simulink model "RCAMSimulation"  (R2020b)
settings: Solver=VariableStepAuto  StartTime=0.0  StopTime=TF  RelTol=1e-3
values from neighbouring files (symbols this model uses):
  u1max = 25*pi/180    (= 0.436332312999)    [InitializeConstants.m]
  u1min = -25*pi/180    (= -0.436332312999)    [InitializeConstants.m]
  u2max = 10*pi/180    (= 0.174532925199)    [InitializeConstants.m]
  u2min = -25*pi/180    (= -0.436332312999)    [InitializeConstants.m]
  u3max = 30*pi/180    (= 0.523598775598)    [InitializeConstants.m]
  u3min = -30*pi/180    (= -0.523598775598)    [InitializeConstants.m]
  u4max = 10*pi/180    (= 0.174532925199)    [InitializeConstants.m]
  u4min = 0.5*pi/180    (= 0.00872664625997)    [InitializeConstants.m]
  u5max = 10*pi/180    (= 0.174532925199)    [InitializeConstants.m]
  u5min = 0.5*pi/180    (= 0.00872664625997)    [InitializeConstants.m]
  x0 = [85 ... (first row only)    [InitializeConstants.m]
undefined symbols (not defined in the file or in its folder): Earth, RCAM_model, WGS84
libraries: aerolibutil x2, aerolibtransform2 x1, aerolibfltsims x1, vrlib x1
settings Model: Creator=admin  LastModifiedBy=Markus

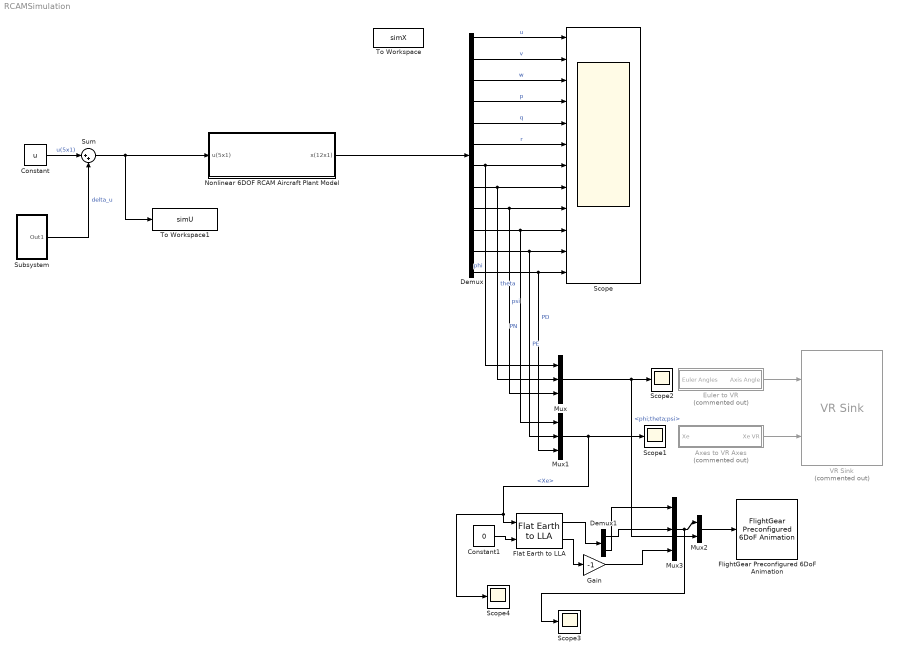
== system RCAMSimulation ==
  Axes to VR Axes : Subsystem  Commented=on
  Constant : Constant  Value=u
  Constant1 : Constant  Value=0
  Demux : Demux  Outputs=12
  Demux1 : Demux  Outputs=2
  Euler to VR : Subsystem  Commented=on
  Flat Earth to LLA : aerolibtransform2/Flat Earth to LLA  units=Metric (MKS)  ptype=Earth (WGS84)  F=1/298.257223563  R=6378137  refPosPort=off  LL0=[0 10]  psi=0
  FlightGear Preconfigured 6DoF Animation : aerolibfltsims/FlightGear Preconfigured 6DoF Animation  xFlightGearVersion=v2019.1  DestinationIpAddress=127.0.0.1  DestinationPort=5502  SampleTime=1/30  packetVersion=24
  Gain : Gain  Gain=-1
  Mux : Mux  Inputs=3
  Mux1 : Mux  Inputs=3
  Mux2 : Mux  Inputs=2
  Mux3 : Mux  Inputs=3
  Nonlinear 6DOF RCAM Aircraft Plant Model : Subsystem
  Scope : Scope  NumInputPorts=12
  Scope{1..4} (4 alike) : Scope
  Subsystem : Subsystem
  Sum : Sum  Inputs=|++
  To Workspace : ToWorkspace  VariableName=simX  SaveFormat=Timeseries  SampleTime=-1
  To Workspace1 : ToWorkspace  VariableName=simU  SaveFormat=Timeseries  SampleTime=-1
  VR Sink : vrlib/VR Sink  Commented=on  InstantiateOnLoad=on  SampleTime=0.1  ViewEnable=on  RemoteChange=off  RemoteView=off  FieldsWritten=HL20.rotation.4.1.1.double#HL20.translation.3.1.1.double  WorldFileName=aeroblk_HL20.wrl  WorldDescription=aeroblk_HL20  AutoView=on  VideoDimensions=[]  AllowVariableSize=off
  wires:
  Nonlinear 6DOF RCAM Aircraft Plant Model/1(x(12x1)) -> Demux/1
  Constant/1 -> Sum/1  "u(5x1)"
  Subsystem/1(Out1) -> Sum/2  "delta_u"
  Sum/1 -> To Workspace1/1, Nonlinear 6DOF RCAM Aircraft Plant Model/1(u(5x1))
  Demux/1 -> Scope/1  "u"
  Demux/2 -> Scope/2  "v"
  Demux/3 -> Scope/3  "w"
  Demux/4 -> Scope/4  "p"
  Demux/5 -> Scope/5  "q"
  Demux/6 -> Scope/6  "r"
  Demux/7 -> Mux/1, Scope/7  "phi"
  Demux/8 -> Mux/2, Scope/8  "theta"
  Demux/9 -> Mux/3, Scope/9  "psi"
  Demux/10 -> Mux1/1, Scope/10  "PN"
  Demux/11 -> Mux1/2, Scope/11  "PE"
  Demux/12 -> Mux1/3, Scope/12  "PD"
  Euler to VR/1(Axis Angle) -> VR Sink/1
  Mux1/1 -> Scope4/1, Flat Earth to LLA/1, Scope1/1  "<Xe>"
  Axes to VR Axes/1(Xe VR) -> VR Sink/2
  Mux/1 -> Mux2/2, Scope2/1  "<phi;theta;psi>"
  Constant1/1 -> Flat Earth to LLA/2
  Mux2/1 -> FlightGear Preconfigured 6DoF Animation/1
  Flat Earth to LLA/1 -> Demux1/1
  Mux3/1 -> Scope3/1, Mux2/1
  Demux1/1 -> Mux3/2
  Flat Earth to LLA/2 -> Gain/1
  Demux1/2 -> Mux3/1
  Gain/1 -> Mux3/3

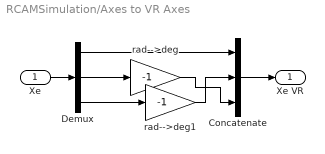
== system RCAMSimulation/Axes to VR Axes ==
  Xe : Inport
  Concatenate : Concatenate  NumInputs=3
  Demux : Demux  Outputs=3
      settings: DisplayOption=none
  rad-->deg : Gain  Gain=-1  SaturateOnIntegerOverflow=on  OutDataTypeStr=Inherit: Same as input  ParamDataTypeStr=Inherit: Same as input
  rad-->deg1 : Gain  Gain=-1  SaturateOnIntegerOverflow=on  OutDataTypeStr=Inherit: Same as input  ParamDataTypeStr=Inherit: Same as input
  Xe VR : Outport  VectorParamsAs1DForOutWhenUnconnected=off
  wires:
  Xe/1 -> Demux/1
  Demux/1 -> Concatenate/1
  Demux/2 -> rad-->deg/1
  Demux/3 -> rad-->deg1/1
  Concatenate/1 -> Xe VR/1
  rad-->deg1/1 -> Concatenate/2
  rad-->deg/1 -> Concatenate/3

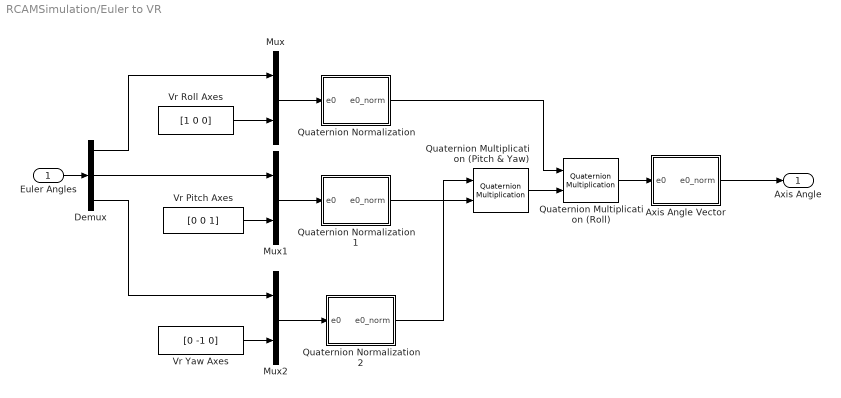
== system RCAMSimulation/Euler to VR ==
  Euler Angles : Inport
  Axis Angle Vector : Subsystem
  Demux : Demux  Outputs=3
      settings: DisplayOption=none
  Mux : Mux  Inputs=2
  Mux1 : Mux  Inputs=2
  Mux2 : Mux  Inputs=2
  Quaternion Multiplication (Pitch & Yaw) : aerolibutil/Quaternion Multiplication
  Quaternion Multiplication (Roll) : aerolibutil/Quaternion Multiplication
  Quaternion Normalization : Subsystem
  Quaternion Normalization1 : Subsystem
  Quaternion Normalization2 : Subsystem
  Vr Pitch Axes : Constant  Value=[0 0 1]
  Vr Roll Axes : Constant  Value=[1 0 0]
  Vr Yaw Axes : Constant  Value=[0 -1 0]
  Axis Angle : Outport  VectorParamsAs1DForOutWhenUnconnected=off
  wires:
  Quaternion Multiplication (Roll)/1 -> Axis Angle Vector/1(e0)
  Quaternion Multiplication (Pitch & Yaw)/1 -> Quaternion Multiplication (Roll)/2
  Axis Angle Vector/1(e0_norm) -> Axis Angle/1
  Quaternion Normalization/1(e0_norm) -> Quaternion Multiplication (Roll)/1
  Quaternion Normalization2/1(e0_norm) -> Quaternion Multiplication (Pitch & Yaw)/1
  Quaternion Normalization1/1(e0_norm) -> Quaternion Multiplication (Pitch & Yaw)/2
  Mux2/1 -> Quaternion Normalization2/1(e0)
  Mux1/1 -> Quaternion Normalization1/1(e0)
  Mux/1 -> Quaternion Normalization/1(e0)
  Demux/3 -> Mux2/1
  Vr Yaw Axes/1 -> Mux2/2
  Demux/2 -> Mux1/1
  Vr Pitch Axes/1 -> Mux1/2
  Demux/1 -> Mux/1
  Vr Roll Axes/1 -> Mux/2
  Euler Angles/1 -> Demux/1

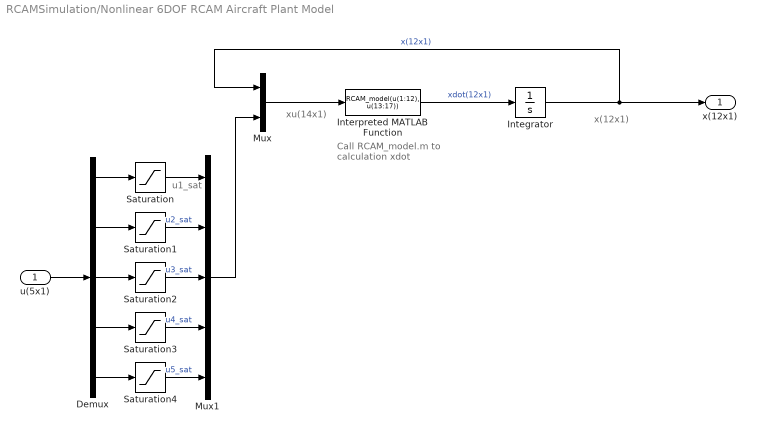
== system RCAMSimulation/Nonlinear 6DOF RCAM Aircraft Plant Model ==
  note: u1_sat
  note: xu(14x1)
  note: x(12x1)
  note: Call RCAM_model.m
      | to calculation xdot
  u(5x1) : Inport
  Demux : Demux  Outputs=5
  Integrator : Integrator  InitialCondition=x0
  Interpreted MATLAB Function : MATLABFcn  MATLABFcn=RCAM_model(u(1:12), u(13:17))
  Mux : Mux  Inputs=2
  Mux1 : Mux  Inputs=5
  Saturation : Saturate  UpperLimit=u1max  LowerLimit=u1min
  Saturation1 : Saturate  UpperLimit=u2max  LowerLimit=u2min
  Saturation2 : Saturate  UpperLimit=u3max  LowerLimit=u3min
  Saturation3 : Saturate  UpperLimit=u4max  LowerLimit=u4min
  Saturation4 : Saturate  UpperLimit=u5max  LowerLimit=u5min
  x(12x1) : Outport
  wires:
  Integrator/1 -> x(12x1)/1, Mux/1  "x(12x1)"
  u(5x1)/1 -> Demux/1
  Interpreted MATLAB Function/1 -> Integrator/1  "xdot(12x1)"
  Mux/1 -> Interpreted MATLAB Function/1
  Demux/1 -> Saturation/1
  Saturation/1 -> Mux1/1
  Demux/2 -> Saturation1/1
  Saturation1/1 -> Mux1/2  "u2_sat"
  Demux/3 -> Saturation2/1
  Saturation2/1 -> Mux1/3  "u3_sat"
  Demux/4 -> Saturation3/1
  Saturation3/1 -> Mux1/4  "u4_sat"
  Demux/5 -> Saturation4/1
  Saturation4/1 -> Mux1/5  "u5_sat"
  Mux1/1 -> Mux/2

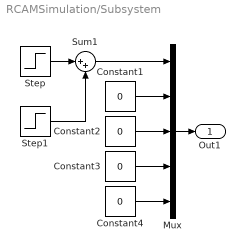
== system RCAMSimulation/Subsystem ==
  Constant{1..4} (4 alike) : Constant  Value=0
  Mux : Mux  Inputs=5
  Step : Step  Time=30  After=5*pi/180  SampleTime=0
  Step1 : Step  Time=30+2  After=-5*pi/180  SampleTime=0
  Sum1 : Sum  Inputs=|++
  Out1 : Outport
  wires:
  Constant2/1 -> Mux/3
  Step1/1 -> Sum1/2
  Constant3/1 -> Mux/4
  Mux/1 -> Out1/1
  Sum1/1 -> Mux/1
  Step/1 -> Sum1/1
  Constant4/1 -> Mux/5
  Constant1/1 -> Mux/2

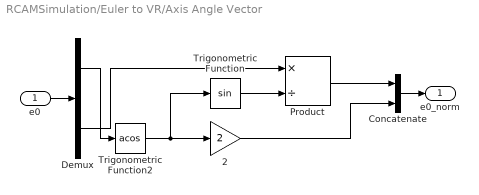
== system RCAMSimulation/Euler to VR/Axis Angle Vector ==
  e0 : Inport
  2 : Gain  Gain=2  SaturateOnIntegerOverflow=on  OutDataTypeStr=Inherit: Same as input  ParamDataTypeStr=Inherit: Same as input
  Concatenate : Concatenate
  Demux : Demux  Outputs=[1 3 ]
      settings: DisplayOption=none
  Product : Product  Inputs=*/  InputSameDT=on  SaturateOnIntegerOverflow=on  OutDataTypeStr=Inherit: Same as first input
  Trigonometric Function : Trigonometry
  Trigonometric Function2 : Trigonometry  Operator=acos
  e0_norm : Outport  VectorParamsAs1DForOutWhenUnconnected=off
  wires:
  Demux/1 -> Trigonometric Function2/1
  Demux/2 -> Product/1
  Concatenate/1 -> e0_norm/1
  Product/1 -> Concatenate/1
  2/1 -> Concatenate/2
  Trigonometric Function/1 -> Product/2
  Trigonometric Function2/1 -> Trigonometric Function/1, 2/1
  e0/1 -> Demux/1

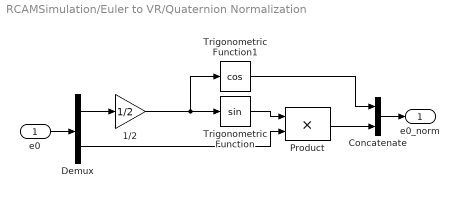
== system RCAMSimulation/Euler to VR/Quaternion Normalization ==
  e0 : Inport
  1/2 : Gain  Gain=1/2  SaturateOnIntegerOverflow=on  OutDataTypeStr=Inherit: Same as input  ParamDataTypeStr=Inherit: Same as input
  Concatenate : Concatenate
  Demux : Demux  Outputs=[1 3]
      settings: DisplayOption=none
  Product : Product  InputSameDT=on  SaturateOnIntegerOverflow=on  OutDataTypeStr=Inherit: Same as first input
  Trigonometric Function : Trigonometry
  Trigonometric Function1 : Trigonometry  Operator=cos
  e0_norm : Outport  VectorParamsAs1DForOutWhenUnconnected=off
  wires:
  Trigonometric Function1/1 -> Concatenate/1
  Demux/2 -> Product/2
  Demux/1 -> 1/2/1
  Concatenate/1 -> e0_norm/1
  Product/1 -> Concatenate/2
  Trigonometric Function/1 -> Product/1
  1/2/1 -> Trigonometric Function1/1, Trigonometric Function/1
  e0/1 -> Demux/1

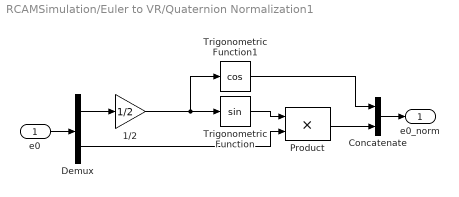
== system RCAMSimulation/Euler to VR/Quaternion Normalization1 ==
  e0 : Inport
  1/2 : Gain  Gain=1/2  SaturateOnIntegerOverflow=on  OutDataTypeStr=Inherit: Same as input  ParamDataTypeStr=Inherit: Same as input
  Concatenate : Concatenate
  Demux : Demux  Outputs=[1 3]
      settings: DisplayOption=none
  Product : Product  InputSameDT=on  SaturateOnIntegerOverflow=on  OutDataTypeStr=Inherit: Same as first input
  Trigonometric Function : Trigonometry
  Trigonometric Function1 : Trigonometry  Operator=cos
  e0_norm : Outport  VectorParamsAs1DForOutWhenUnconnected=off
  wires:
  e0/1 -> Demux/1
  1/2/1 -> Trigonometric Function/1, Trigonometric Function1/1
  Trigonometric Function/1 -> Product/1
  Product/1 -> Concatenate/2
  Concatenate/1 -> e0_norm/1
  Demux/1 -> 1/2/1
  Demux/2 -> Product/2
  Trigonometric Function1/1 -> Concatenate/1

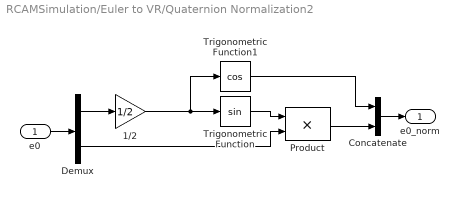
== system RCAMSimulation/Euler to VR/Quaternion Normalization2 ==
  e0 : Inport
  1/2 : Gain  Gain=1/2  SaturateOnIntegerOverflow=on  OutDataTypeStr=Inherit: Same as input  ParamDataTypeStr=Inherit: Same as input
  Concatenate : Concatenate
  Demux : Demux  Outputs=[1 3]
      settings: DisplayOption=none
  Product : Product  InputSameDT=on  SaturateOnIntegerOverflow=on  OutDataTypeStr=Inherit: Same as first input
  Trigonometric Function : Trigonometry
  Trigonometric Function1 : Trigonometry  Operator=cos
  e0_norm : Outport  VectorParamsAs1DForOutWhenUnconnected=off
  wires:
  Trigonometric Function1/1 -> Concatenate/1
  Demux/2 -> Product/2
  Demux/1 -> 1/2/1
  Concatenate/1 -> e0_norm/1
  Product/1 -> Concatenate/2
  Trigonometric Function/1 -> Product/1
  1/2/1 -> Trigonometric Function1/1, Trigonometric Function/1
  e0/1 -> Demux/1
